simulink library "dlbsBlockSumOverMultipleDimensions"  (R2025b)
settings: Solver=VariableStepAuto  StartTime=0.0  StopTime=10.0  RelTol=1e-3
settings Model: Creator=lt6037  LastModifiedBy=lt6037

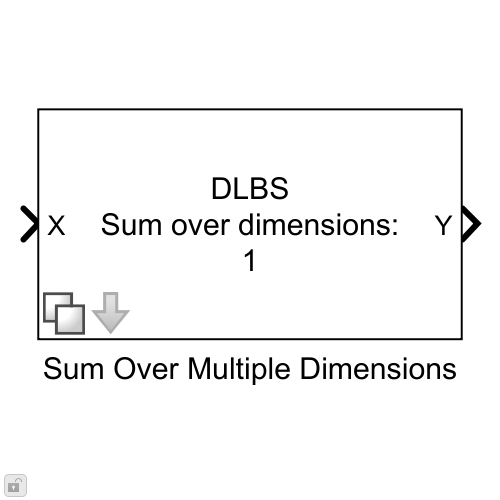
[thumbnail: Simulink's stored preview of the top-level diagram]
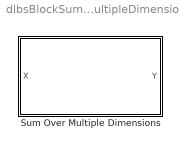
== system dlbsBlockSumOverMultipleDimensions ==
  Sum Over Multiple Dimensions : Subsystem  Variant=on  PassThrough=on  AllowFlexibleInterface=off  mask{dims=1}
      mask prompts: dims "Dimensions to sum over"
      mask help:
      | Sums an input tensor over a user-defined set of dimensions.
      | This block is a no-gradient operation and does not pass gradients back.
      mask Help: web("dlbsHelpBlockSumOverMultipleDimensions.html")
      mask Display:
      | %ws = Simulink.Mask.get(gcbh).getWorkspace();
      | fprintf("DLBS\nSum over dimensions:\n%s",get_param(gcbh,"dims"))

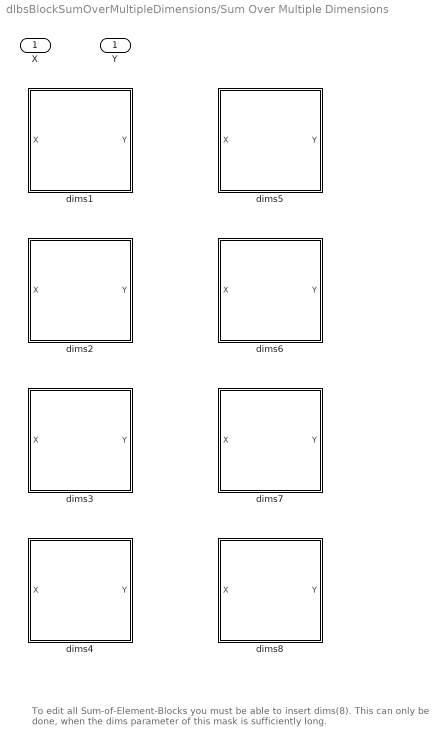
== system dlbsBlockSumOverMultipleDimensions/Sum Over Multiple Dimensions ==
  note: To edit all Sum-of-Element-Blocks you must be able to insert dims(8).
      | This can only be done, when the dims parameter of this mask is sufficiently long.
  X : Inport
  dims1 : Subsystem  VariantControl=length_dims==1
      mask help: Default Mask
  dims2 : Subsystem  VariantControl=length_dims==2
      mask help: Default Mask
  dims3 : Subsystem  VariantControl=length_dims==3
      mask help: Default Mask
  dims4 : Subsystem  VariantControl=length_dims==4
      mask help: Default Mask
  dims5 : Subsystem  VariantControl=length_dims==5
      mask help: Default Mask
  dims6 : Subsystem  VariantControl=length_dims==6
      mask help: Default Mask
  dims7 : Subsystem  VariantControl=length_dims==7
      mask help: Default Mask
  dims8 : Subsystem  VariantControl=length_dims==8
      mask help: Default Mask
  Y : Outport

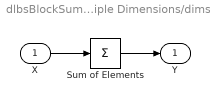
== system dlbsBlockSumOverMultipleDimensions/Sum Over Multiple Dimensions/dims1 ==
  X : Inport
  Sum of Elements : Sum  Inputs=+  CollapseMode=Specified dimension  CollapseDim=dims(1)
      settings: AttributesFormatString=%<CollapseDim>
  Y : Outport
  wires:
  X/1 -> Sum of Elements/1
  Sum of Elements/1 -> Y/1

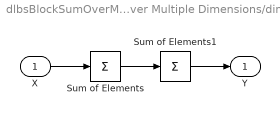
== system dlbsBlockSumOverMultipleDimensions/Sum Over Multiple Dimensions/dims2 ==
  X : Inport
  Sum of Elements : Sum  Inputs=+  CollapseMode=Specified dimension  CollapseDim=dims(1)
      settings: AttributesFormatString=%<CollapseDim>
  Sum of Elements1 : Sum  Inputs=+  CollapseMode=Specified dimension  CollapseDim=dims(2)
      settings: AttributesFormatString=%<CollapseDim>
  Y : Outport
  wires:
  Sum of Elements1/1 -> Y/1
  X/1 -> Sum of Elements/1
  Sum of Elements/1 -> Sum of Elements1/1

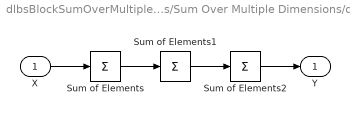
== system dlbsBlockSumOverMultipleDimensions/Sum Over Multiple Dimensions/dims3 ==
  X : Inport
  Sum of Elements : Sum  Inputs=+  CollapseMode=Specified dimension  CollapseDim=dims(1)
      settings: AttributesFormatString=%<CollapseDim>
  Sum of Elements1 : Sum  Inputs=+  CollapseMode=Specified dimension  CollapseDim=dims(2)
      settings: AttributesFormatString=%<CollapseDim>
  Sum of Elements2 : Sum  Inputs=+  CollapseMode=Specified dimension  CollapseDim=dims(3)
      settings: AttributesFormatString=%<CollapseDim>
  Y : Outport
  wires:
  X/1 -> Sum of Elements/1
  Sum of Elements/1 -> Sum of Elements1/1
  Sum of Elements1/1 -> Sum of Elements2/1
  Sum of Elements2/1 -> Y/1

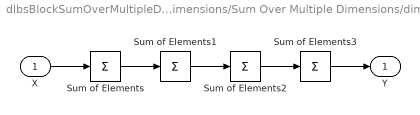
== system dlbsBlockSumOverMultipleDimensions/Sum Over Multiple Dimensions/dims4 ==
  X : Inport
  Sum of Elements : Sum  Inputs=+  CollapseMode=Specified dimension  CollapseDim=dims(1)
      settings: AttributesFormatString=%<CollapseDim>
  Sum of Elements1 : Sum  Inputs=+  CollapseMode=Specified dimension  CollapseDim=dims(2)
      settings: AttributesFormatString=%<CollapseDim>
  Sum of Elements2 : Sum  Inputs=+  CollapseMode=Specified dimension  CollapseDim=dims(3)
      settings: AttributesFormatString=%<CollapseDim>
  Sum of Elements3 : Sum  Inputs=+  CollapseMode=Specified dimension  CollapseDim=dims(4)
      settings: AttributesFormatString=%<CollapseDim>
  Y : Outport
  wires:
  Sum of Elements3/1 -> Y/1
  X/1 -> Sum of Elements/1
  Sum of Elements/1 -> Sum of Elements1/1
  Sum of Elements2/1 -> Sum of Elements3/1
  Sum of Elements1/1 -> Sum of Elements2/1

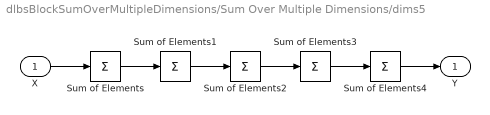
== system dlbsBlockSumOverMultipleDimensions/Sum Over Multiple Dimensions/dims5 ==
  X : Inport
  Sum of Elements : Sum  Inputs=+  CollapseMode=Specified dimension  CollapseDim=dims(1)
      settings: AttributesFormatString=%<CollapseDim>
  Sum of Elements1 : Sum  Inputs=+  CollapseMode=Specified dimension  CollapseDim=dims(2)
      settings: AttributesFormatString=%<CollapseDim>
  Sum of Elements2 : Sum  Inputs=+  CollapseMode=Specified dimension  CollapseDim=dims(3)
      settings: AttributesFormatString=%<CollapseDim>
  Sum of Elements3 : Sum  Inputs=+  CollapseMode=Specified dimension  CollapseDim=dims(4)
      settings: AttributesFormatString=%<CollapseDim>
  Sum of Elements4 : Sum  Inputs=+  CollapseMode=Specified dimension  CollapseDim=dims(5)
      settings: AttributesFormatString=%<CollapseDim>
  Y : Outport
  wires:
  Sum of Elements4/1 -> Y/1
  X/1 -> Sum of Elements/1
  Sum of Elements2/1 -> Sum of Elements3/1
  Sum of Elements/1 -> Sum of Elements1/1
  Sum of Elements1/1 -> Sum of Elements2/1
  Sum of Elements3/1 -> Sum of Elements4/1

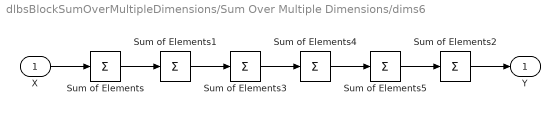
== system dlbsBlockSumOverMultipleDimensions/Sum Over Multiple Dimensions/dims6 ==
  X : Inport
  Sum of Elements : Sum  Inputs=+  CollapseMode=Specified dimension  CollapseDim=dims(1)
      settings: AttributesFormatString=%<CollapseDim>
  Sum of Elements1 : Sum  Inputs=+  CollapseMode=Specified dimension  CollapseDim=dims(2)
      settings: AttributesFormatString=%<CollapseDim>
  Sum of Elements2 : Sum  Inputs=+  CollapseMode=Specified dimension  CollapseDim=dims(6)
      settings: AttributesFormatString=%<CollapseDim>
  Sum of Elements3 : Sum  Inputs=+  CollapseMode=Specified dimension  CollapseDim=dims(3)
      settings: AttributesFormatString=%<CollapseDim>
  Sum of Elements4 : Sum  Inputs=+  CollapseMode=Specified dimension  CollapseDim=dims(4)
      settings: AttributesFormatString=%<CollapseDim>
  Sum of Elements5 : Sum  Inputs=+  CollapseMode=Specified dimension  CollapseDim=dims(5)
      settings: AttributesFormatString=%<CollapseDim>
  Y : Outport
  wires:
  Sum of Elements5/1 -> Sum of Elements2/1
  Sum of Elements1/1 -> Sum of Elements3/1
  X/1 -> Sum of Elements/1
  Sum of Elements3/1 -> Sum of Elements4/1
  Sum of Elements/1 -> Sum of Elements1/1
  Sum of Elements4/1 -> Sum of Elements5/1
  Sum of Elements2/1 -> Y/1

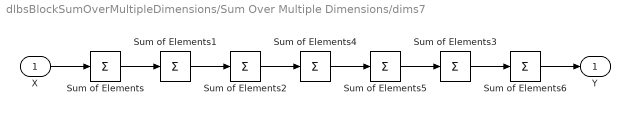
== system dlbsBlockSumOverMultipleDimensions/Sum Over Multiple Dimensions/dims7 ==
  X : Inport
  Sum of Elements : Sum  Inputs=+  CollapseMode=Specified dimension  CollapseDim=dims(1)
      settings: AttributesFormatString=%<CollapseDim>
  Sum of Elements1 : Sum  Inputs=+  CollapseMode=Specified dimension  CollapseDim=dims(2)
      settings: AttributesFormatString=%<CollapseDim>
  Sum of Elements2 : Sum  Inputs=+  CollapseMode=Specified dimension  CollapseDim=dims(3)
      settings: AttributesFormatString=%<CollapseDim>
  Sum of Elements3 : Sum  Inputs=+  CollapseMode=Specified dimension  CollapseDim=dims(6)
      settings: AttributesFormatString=%<CollapseDim>
  Sum of Elements4 : Sum  Inputs=+  CollapseMode=Specified dimension  CollapseDim=dims(4)
      settings: AttributesFormatString=%<CollapseDim>
  Sum of Elements5 : Sum  Inputs=+  CollapseMode=Specified dimension  CollapseDim=dims(5)
      settings: AttributesFormatString=%<CollapseDim>
  Sum of Elements6 : Sum  Inputs=+  CollapseMode=Specified dimension  CollapseDim=dims(7)
      settings: AttributesFormatString=%<CollapseDim>
  Y : Outport
  wires:
  Sum of Elements2/1 -> Sum of Elements4/1
  X/1 -> Sum of Elements/1
  Sum of Elements4/1 -> Sum of Elements5/1
  Sum of Elements/1 -> Sum of Elements1/1
  Sum of Elements3/1 -> Sum of Elements6/1
  Sum of Elements1/1 -> Sum of Elements2/1
  Sum of Elements5/1 -> Sum of Elements3/1
  Sum of Elements6/1 -> Y/1

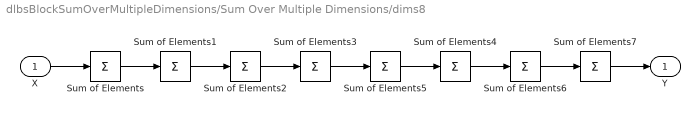
== system dlbsBlockSumOverMultipleDimensions/Sum Over Multiple Dimensions/dims8 ==
  X : Inport
  Sum of Elements : Sum  Inputs=+  CollapseMode=Specified dimension  CollapseDim=dims(1)
      settings: AttributesFormatString=%<CollapseDim>
  Sum of Elements1 : Sum  Inputs=+  CollapseMode=Specified dimension  CollapseDim=dims(2)
      settings: AttributesFormatString=%<CollapseDim>
  Sum of Elements2 : Sum  Inputs=+  CollapseMode=Specified dimension  CollapseDim=dims(3)
      settings: AttributesFormatString=%<CollapseDim>
  Sum of Elements3 : Sum  Inputs=+  CollapseMode=Specified dimension  CollapseDim=dims(4)
      settings: AttributesFormatString=%<CollapseDim>
  Sum of Elements4 : Sum  Inputs=+  CollapseMode=Specified dimension  CollapseDim=dims(6)
      settings: AttributesFormatString=%<CollapseDim>
  Sum of Elements5 : Sum  Inputs=+  CollapseMode=Specified dimension  CollapseDim=dims(5)
      settings: AttributesFormatString=%<CollapseDim>
  Sum of Elements6 : Sum  Inputs=+  CollapseMode=Specified dimension  CollapseDim=dims(7)
      settings: AttributesFormatString=%<CollapseDim>
  Sum of Elements7 : Sum  Inputs=+  CollapseMode=Specified dimension  CollapseDim=dims(8)
      settings: AttributesFormatString=%<CollapseDim>
  Y : Outport
  wires:
  Sum of Elements2/1 -> Sum of Elements3/1
  X/1 -> Sum of Elements/1
  Sum of Elements3/1 -> Sum of Elements5/1
  Sum of Elements/1 -> Sum of Elements1/1
  Sum of Elements7/1 -> Y/1
  Sum of Elements1/1 -> Sum of Elements2/1
  Sum of Elements4/1 -> Sum of Elements6/1
  Sum of Elements5/1 -> Sum of Elements4/1
  Sum of Elements6/1 -> Sum of Elements7/1
